simulink library "ESTS_VVSO"  (R2024b)
settings: Solver=VariableStepAuto  StartTime=0.0  StopTime=10.0  RelTol=1e-3
libraries: ESTS_VVSO_WHL x1
settings Model: Creator=blatak  LastModifiedBy=blatak
settings ModelReferenceCC: EnableRefExpFcnMdlSchedulingChecks=on
settings RTWCC: GPUComputeCapability=3.5

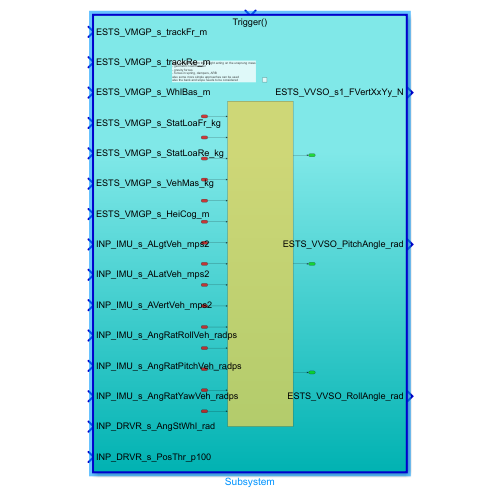
[thumbnail: Simulink's stored preview of the top-level diagram]
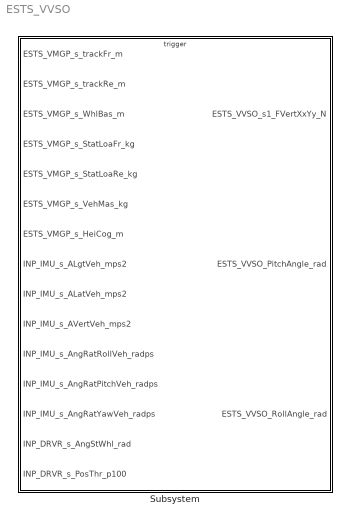
== system ESTS_VVSO ==
  Subsystem : Subsystem

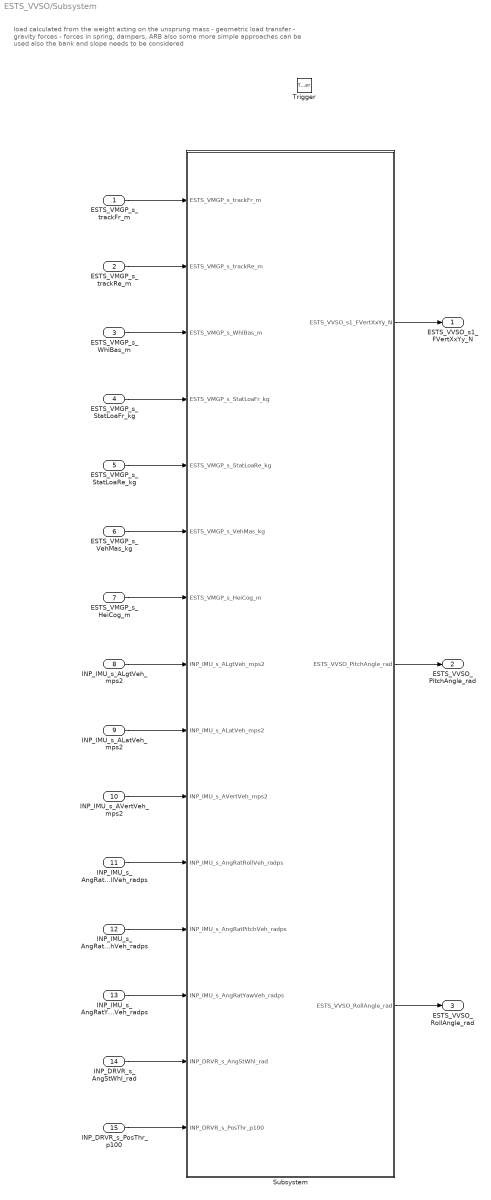
== system ESTS_VVSO/Subsystem ==
  note: load calculated from the weight acting on the unsprung mass
      | - geometric load transfer
      | - gravity forces
      | - forces in spring, dampers, ARB
      | also some more simple approaches can be used
      | also the bank and slope needs to be considered
  ESTS_VMGP_s_trackFr_m : Inport
  ESTS_VMGP_s_trackRe_m : Inport  Port=2
  ESTS_VMGP_s_WhlBas_m : Inport  Port=3
  ESTS_VMGP_s_StatLoaFr_kg : Inport  Port=4
  ESTS_VMGP_s_StatLoaRe_kg : Inport  Port=5
  ESTS_VMGP_s_VehMas_kg : Inport  Port=6
  ESTS_VMGP_s_HeiCog_m : Inport  Port=7
  INP_IMU_s_ALgtVeh_mps2 : Inport  Port=8
  INP_IMU_s_ALatVeh_mps2 : Inport  Port=9
  INP_IMU_s_AVertVeh_mps2 : Inport  Port=10
  INP_IMU_s_AngRatRollVeh_radps : Inport  Port=11
  INP_IMU_s_AngRatPitchVeh_radps : Inport  Port=12
  INP_IMU_s_AngRatYawVeh_radps : Inport  Port=13
  INP_DRVR_s_AngStWhl_rad : Inport  Port=14
  INP_DRVR_s_PosThr_p100 : Inport  Port=15
  Trigger : TriggerPort  TriggerType=function-call  VariantControl=(inherit)  PortDimensions=1
  Subsystem : Subsystem
  ESTS_VVSO_s1_FVertXxYy_N : Outport
  ESTS_VVSO_PitchAngle_rad : Outport  Port=2
  ESTS_VVSO_RollAngle_rad : Outport  Port=3
  wires:
  ESTS_VMGP_s_trackFr_m/1 -> Subsystem/1(ESTS_VMGP_s_trackFr_m)
  ESTS_VMGP_s_trackRe_m/1 -> Subsystem/2(ESTS_VMGP_s_trackRe_m)
  ESTS_VMGP_s_WhlBas_m/1 -> Subsystem/3(ESTS_VMGP_s_WhlBas_m)
  ESTS_VMGP_s_StatLoaFr_kg/1 -> Subsystem/4(ESTS_VMGP_s_StatLoaFr_kg)
  ESTS_VMGP_s_StatLoaRe_kg/1 -> Subsystem/5(ESTS_VMGP_s_StatLoaRe_kg)
  ESTS_VMGP_s_VehMas_kg/1 -> Subsystem/6(ESTS_VMGP_s_VehMas_kg)
  ESTS_VMGP_s_HeiCog_m/1 -> Subsystem/7(ESTS_VMGP_s_HeiCog_m)
  INP_IMU_s_ALgtVeh_mps2/1 -> Subsystem/8(INP_IMU_s_ALgtVeh_mps2)
  INP_IMU_s_ALatVeh_mps2/1 -> Subsystem/9(INP_IMU_s_ALatVeh_mps2)
  INP_IMU_s_AVertVeh_mps2/1 -> Subsystem/10(INP_IMU_s_AVertVeh_mps2)
  INP_IMU_s_AngRatRollVeh_radps/1 -> Subsystem/11(INP_IMU_s_AngRatRollVeh_radps)
  INP_IMU_s_AngRatPitchVeh_radps/1 -> Subsystem/12(INP_IMU_s_AngRatPitchVeh_radps)
  INP_IMU_s_AngRatYawVeh_radps/1 -> Subsystem/13(INP_IMU_s_AngRatYawVeh_radps)
  INP_DRVR_s_AngStWhl_rad/1 -> Subsystem/14(INP_DRVR_s_AngStWhl_rad)
  INP_DRVR_s_PosThr_p100/1 -> Subsystem/15(INP_DRVR_s_PosThr_p100)
  Subsystem/1(ESTS_VVSO_s1_FVertXxYy_N) -> ESTS_VVSO_s1_FVertXxYy_N/1
  Subsystem/2(ESTS_VVSO_PitchAngle_rad) -> ESTS_VVSO_PitchAngle_rad/1
  Subsystem/3(ESTS_VVSO_RollAngle_rad) -> ESTS_VVSO_RollAngle_rad/1

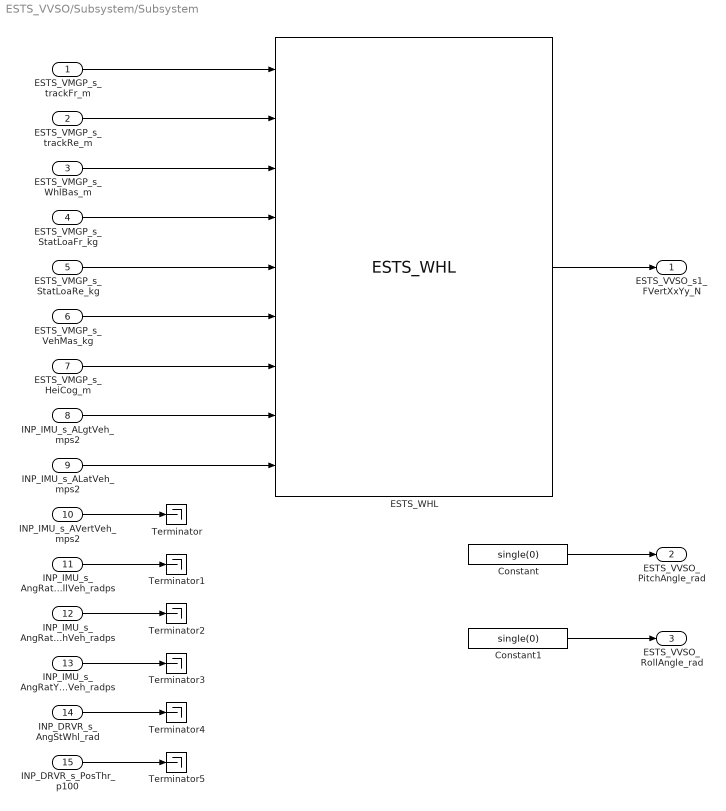
== system ESTS_VVSO/Subsystem/Subsystem ==
  ESTS_VMGP_s_trackFr_m : Inport
  ESTS_VMGP_s_trackRe_m : Inport  Port=2
  ESTS_VMGP_s_WhlBas_m : Inport  Port=3
  ESTS_VMGP_s_StatLoaFr_kg : Inport  Port=4
  ESTS_VMGP_s_StatLoaRe_kg : Inport  Port=5
  ESTS_VMGP_s_VehMas_kg : Inport  Port=6
  ESTS_VMGP_s_HeiCog_m : Inport  Port=7
  INP_IMU_s_ALgtVeh_mps2 : Inport  Port=8
  INP_IMU_s_ALatVeh_mps2 : Inport  Port=9
  INP_IMU_s_AVertVeh_mps2 : Inport  Port=10
  INP_IMU_s_AngRatRollVeh_radps : Inport  Port=11
  INP_IMU_s_AngRatPitchVeh_radps : Inport  Port=12
  INP_IMU_s_AngRatYawVeh_radps : Inport  Port=13
  INP_DRVR_s_AngStWhl_rad : Inport  Port=14
  INP_DRVR_s_PosThr_p100 : Inport  Port=15
  Constant : Constant  Value=single(0)
  Constant1 : Constant  Value=single(0)
  ESTS_WHL : ESTS_VVSO_WHL/ESTS_WHL  SystemSampleTime=-1  VariantActivationTime=update diagram  AllowFlexibleInterface=on  Latency=0  AutoFrameSizeCalculation=off
  Terminator{,1..5} (6 alike) : Terminator
  ESTS_VVSO_s1_FVertXxYy_N : Outport
  ESTS_VVSO_PitchAngle_rad : Outport  Port=2
  ESTS_VVSO_RollAngle_rad : Outport  Port=3
  wires:
  ESTS_WHL/1 -> ESTS_VVSO_s1_FVertXxYy_N/1
  ESTS_VMGP_s_trackFr_m/1 -> ESTS_WHL/1
  ESTS_VMGP_s_trackRe_m/1 -> ESTS_WHL/2
  ESTS_VMGP_s_WhlBas_m/1 -> ESTS_WHL/3
  ESTS_VMGP_s_StatLoaFr_kg/1 -> ESTS_WHL/4
  ESTS_VMGP_s_StatLoaRe_kg/1 -> ESTS_WHL/5
  ESTS_VMGP_s_VehMas_kg/1 -> ESTS_WHL/6
  ESTS_VMGP_s_HeiCog_m/1 -> ESTS_WHL/7
  INP_IMU_s_ALgtVeh_mps2/1 -> ESTS_WHL/8
  INP_IMU_s_ALatVeh_mps2/1 -> ESTS_WHL/9
  Constant/1 -> ESTS_VVSO_PitchAngle_rad/1
  Constant1/1 -> ESTS_VVSO_RollAngle_rad/1
  INP_DRVR_s_PosThr_p100/1 -> Terminator5/1
  INP_DRVR_s_AngStWhl_rad/1 -> Terminator4/1
  INP_IMU_s_AngRatYawVeh_radps/1 -> Terminator3/1
  INP_IMU_s_AngRatPitchVeh_radps/1 -> Terminator2/1
  INP_IMU_s_AngRatRollVeh_radps/1 -> Terminator1/1
  INP_IMU_s_AVertVeh_mps2/1 -> Terminator/1
